simulink subsystem "rss_ClarkeTrasf"  (R2023a)
settings: Solver=VariableStepAuto  StartTime=0.0  StopTime=inf  RelTol=1e-3
undefined symbols (not defined in the file): Cdbl_dcycDycMaxVal, Cdbl_iPhCurrMaxVal, Cdbl_nElecAgSpdMaxVal, Cdbl_nElecAgSpdPeakVal, Cdbl_uSplyVltgMaxVal, Gs16_tiPhVltgAgDel_C
libraries: lib_conversion x4, lib_clarke_transform x2, lib_trigonometric_function x2
settings Model: DefaultTestHarness=rss_ClarkeTransform_thu  Creator=CAV2OFO  LastModifiedBy=xiaoqiang.yuan
settings OptimizationCC: ReuseModelBlockBuffer=off

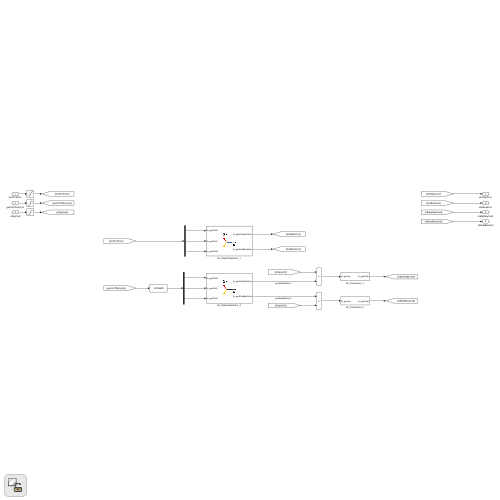
[thumbnail: Simulink's stored preview of the top-level diagram]
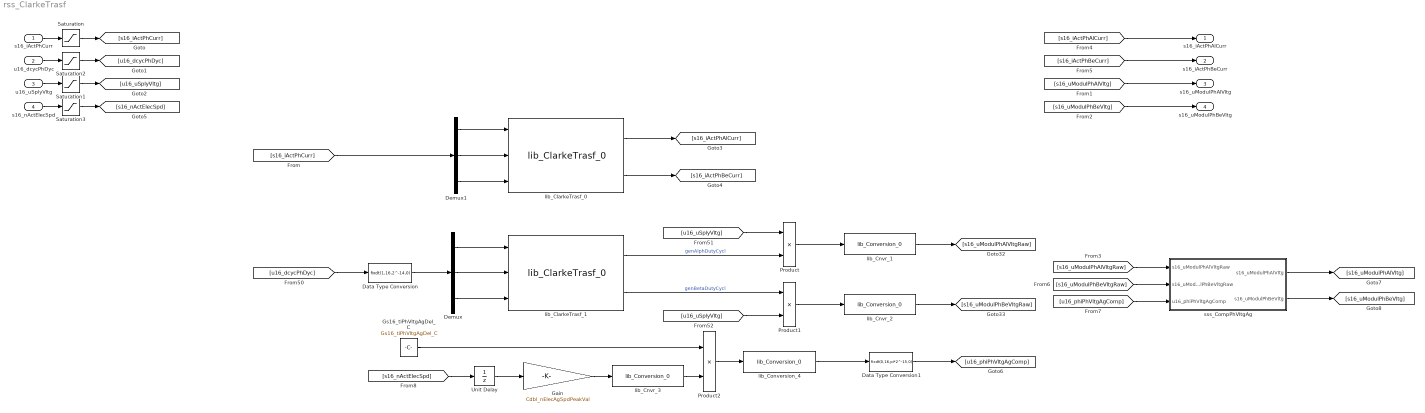
== system rss_ClarkeTrasf ==
  s16_iActPhCurr : Inport  OutDataTypeStr=dt_Standardize_s16p15b0
  u16_dcycPhDyc : Inport  Port=2  OutDataTypeStr=dt_DutyCycl_u16p15b0
  u16_uSplyVltg : Inport  Port=3  OutDataTypeStr=dt_Standardize_u16p15b0
  s16_nActElecSpd : Inport  Port=4  OutDataTypeStr=dt_Standardize_s16p15b0
  Data Type Conversion : DataTypeConversion  OutDataTypeStr=fixdt(1,16,2^-14,0)  SaturateOnIntegerOverflow=off  RndMeth=Floor
  Data Type Conversion1 : DataTypeConversion  OutDataTypeStr=fixdt(0,16,pi*2^-15,0)  SaturateOnIntegerOverflow=off  RndMeth=Floor
  Demux : Demux  Outputs=3
  Demux1 : Demux  Outputs=3
  Gain : Gain  Gain=Cdbl_nElecAgSpdPeakVal  OutDataTypeStr=Inherit: Inherit via back propagation
  Gs16_tiPhVltgAgDel_C : Constant  Value=Gs16_tiPhVltgAgDel_C
  Product : Product  OutDataTypeStr=Inherit: Inherit via back propagation
  Product1 : Product  OutDataTypeStr=Inherit: Inherit via back propagation
  Product2 : Product  OutDataTypeStr=Inherit: Inherit via back propagation
  Saturation : Saturate  UpperLimit=Cdbl_iPhCurrMaxVal  LowerLimit=-Cdbl_iPhCurrMaxVal
  Saturation1 : Saturate  UpperLimit=Cdbl_uSplyVltgMaxVal  LowerLimit=0
  Saturation2 : Saturate  UpperLimit=Cdbl_dcycDycMaxVal  LowerLimit=0
  Saturation3 : Saturate  UpperLimit=Cdbl_nElecAgSpdMaxVal  LowerLimit=-Cdbl_nElecAgSpdMaxVal
  Unit Delay : UnitDelay  SampleTime=-1  HasFrameUpgradeWarning=on
  lib_ClarkeTrasf_0 : lib_clarke_transform/lib_ClarkeTrasf_0  VariantControl=ClarkTransf_MIL_flo  lb_parAccmDataType=fixdt(1,16,2^-14,0)  lb_parUnBalcSys=off
      settings: LibrarySourceBlock=lib_clarke_transform/lib_ClarkeTransform_0
  lib_ClarkeTrasf_1 : lib_clarke_transform/lib_ClarkeTrasf_0  VariantControl=ClarkTransf_MIL_flo  lb_parAccmDataType=fixdt(1,16,2^-13,0)  lb_parUnBalcSys=on
      settings: LibrarySourceBlock=lib_clarke_transform/lib_ClarkeTransform_0
  lib_Cnvr_1 : lib_conversion/lib_Conversion_0  lb_parDataType=dt_Standardize_s16p15b0  lb_parOutpMaxVal=[]  lb_parOutpMinVal=[]  lb_parSatFlag=off
  lib_Cnvr_2 : lib_conversion/lib_Conversion_0  lb_parDataType=dt_Standardize_s16p15b0  lb_parOutpMaxVal=[]  lb_parOutpMinVal=[]  lb_parSatFlag=off
  lib_Cnvr_3 : lib_conversion/lib_Conversion_0  lb_parDataType=fixdt(1,16)  lb_parOutpMaxVal=Cdbl_nElecAgSpdPeakVal  lb_parOutpMinVal=[]  RndMeth=Simplest  lb_parSatFlag=off
  lib_Conversion_4 : lib_conversion/lib_Conversion_0  lb_parDataType=fixdt(1,16,pi*2^-15,0)  lb_parOutpMaxVal=[]  lb_parOutpMinVal=[]  lb_parSatFlag=off
  sss_CompPhVltgAg : Subsystem
  s16_iActPhAlCurr : Outport  OutDataTypeStr=dt_Standardize_s16p15b0
  s16_iActPhBeCurr : Outport  Port=2  OutDataTypeStr=dt_Standardize_s16p15b0
  s16_uModulPhAlVltg : Outport  Port=3  OutDataTypeStr=dt_Standardize_s16p15b0
  s16_uModulPhBeVltg : Outport  Port=4  OutDataTypeStr=dt_Standardize_s16p15b0
  wires:
  Demux1/1 -> lib_ClarkeTrasf_0/1
  Demux1/3 -> lib_ClarkeTrasf_0/3
  Demux1/2 -> lib_ClarkeTrasf_0/2
  s16_iActPhCurr/1 -> Saturation/1
  [s16_iActPhCurr] -> Demux1/1
  [s16_iActPhAlCurr] -> s16_iActPhAlCurr/1
  [s16_iActPhBeCurr] -> s16_iActPhBeCurr/1
  lib_ClarkeTrasf_0/1 -> [s16_iActPhAlCurr]
  lib_ClarkeTrasf_0/2 -> [s16_iActPhBeCurr]
  Saturation/1 -> [s16_iActPhCurr]
  [u16_uSplyVltg] -> Product1/2
  u16_dcycPhDyc/1 -> Saturation2/1
  Product1/1 -> lib_Cnvr_2/1
  lib_Cnvr_1/1 -> [s16_uModulPhAlVltgRaw]
  Demux/2 -> lib_ClarkeTrasf_1/2
  Demux/3 -> lib_ClarkeTrasf_1/3
  Product/1 -> lib_Cnvr_1/1
  [u16_dcycPhDyc] -> Data Type Conversion/1
  lib_ClarkeTrasf_1/1 -> Product/2  "genAlphDutyCycl"
  Demux/1 -> lib_ClarkeTrasf_1/1
  lib_Cnvr_2/1 -> [s16_uModulPhBeVltgRaw]
  [s16_uModulPhBeVltg] -> s16_uModulPhBeVltg/1
  lib_ClarkeTrasf_1/2 -> Product1/1  "genBetaDutyCycl"
  Data Type Conversion/1 -> Demux/1
  [u16_uSplyVltg] -> Product/1
  [s16_uModulPhAlVltg] -> s16_uModulPhAlVltg/1
  u16_uSplyVltg/1 -> Saturation1/1
  Saturation1/1 -> [u16_uSplyVltg]
  Saturation2/1 -> [u16_dcycPhDyc]
  Product2/1 -> lib_Conversion_4/1
  Gs16_tiPhVltgAgDel_C/1 -> Product2/1
  Data Type Conversion1/1 -> [u16_phiPhVltgAgComp]
  [s16_nActElecSpd] -> Unit Delay/1
  lib_Conversion_4/1 -> Data Type Conversion1/1
  Saturation3/1 -> [s16_nActElecSpd]
  s16_nActElecSpd/1 -> Saturation3/1
  Gain/1 -> lib_Cnvr_3/1
  lib_Cnvr_3/1 -> Product2/2
  Unit Delay/1 -> Gain/1
  [s16_uModulPhAlVltgRaw] -> sss_CompPhVltgAg/1(s16_uModulPhAlVltgRaw)
  [s16_uModulPhBeVltgRaw] -> sss_CompPhVltgAg/2(s16_uModulPhBeVltgRaw)
  [u16_phiPhVltgAgComp] -> sss_CompPhVltgAg/3(u16_phiPhVltgAgComp)
  sss_CompPhVltgAg/1(s16_uModulPhAlVltg) -> [s16_uModulPhAlVltg]
  sss_CompPhVltgAg/2(s16_uModulPhBeVltg) -> [s16_uModulPhBeVltg]

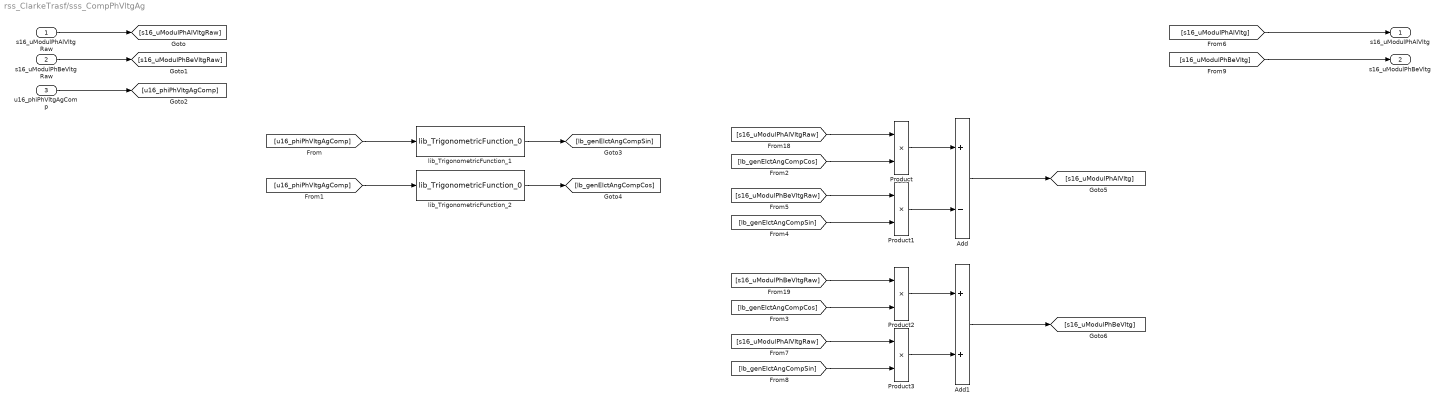
== system rss_ClarkeTrasf/sss_CompPhVltgAg ==
  s16_uModulPhAlVltgRaw : Inport
  s16_uModulPhBeVltgRaw : Inport  Port=2
  u16_phiPhVltgAgComp : Inport  Port=3
  Add : Sum  Inputs=+-  OutDataTypeStr=Inherit: Same as first input
  Add1 : Sum  OutDataTypeStr=Inherit: Same as first input
  Product{,1..3} (4 alike) : Product  OutDataTypeStr=Inherit: Same as first input
  lib_TrigonometricFunction_1 : lib_trigonometric_function/lib_TrigonometricFunction_0  lb_parSelSigType=Sine  lb_parLktSizeStr=1024  lb_parOutpDataType=fixdt(1,16,2^-14,0)
  lib_TrigonometricFunction_2 : lib_trigonometric_function/lib_TrigonometricFunction_0  lb_parSelSigType=Cosine  lb_parLktSizeStr=1024  lb_parOutpDataType=fixdt(1,16,2^-14,0)
  s16_uModulPhAlVltg : Outport
  s16_uModulPhBeVltg : Outport  Port=2
  wires:
  [s16_uModulPhBeVltg] -> s16_uModulPhBeVltg/1
  [s16_uModulPhAlVltg] -> s16_uModulPhAlVltg/1
  Product2/1 -> Add1/1
  [s16_uModulPhBeVltgRaw] -> Product2/1
  Product3/1 -> Add1/2
  Add1/1 -> [s16_uModulPhBeVltg]
  [lb_genElctAngCompSin] -> Product3/2
  [lb_genElctAngCompCos] -> Product2/2
  [s16_uModulPhAlVltgRaw] -> Product3/1
  Add/1 -> [s16_uModulPhAlVltg]
  Product/1 -> Add/1
  Product1/1 -> Add/2
  [s16_uModulPhBeVltgRaw] -> Product1/1
  [lb_genElctAngCompSin] -> Product1/2
  [lb_genElctAngCompCos] -> Product/2
  [s16_uModulPhAlVltgRaw] -> Product/1
  lib_TrigonometricFunction_2/1 -> [lb_genElctAngCompCos]
  lib_TrigonometricFunction_1/1 -> [lb_genElctAngCompSin]
  [u16_phiPhVltgAgComp] -> lib_TrigonometricFunction_2/1
  [u16_phiPhVltgAgComp] -> lib_TrigonometricFunction_1/1
  u16_phiPhVltgAgComp/1 -> [u16_phiPhVltgAgComp]
  s16_uModulPhBeVltgRaw/1 -> [s16_uModulPhBeVltgRaw]
  s16_uModulPhAlVltgRaw/1 -> [s16_uModulPhAlVltgRaw]
